simulink model "Trajectory_Tracking_Car_Backstepping_Algorithm"  (R2022b)
settings: Solver=FixedStepAuto  StartTime=0.0  StopTime=Tf  FixedStep=Ts  RelTol=1e-3
values from neighbouring files (symbols this model uses):
  alpha = 3    [Setup_Trajectory_FL_MPC.m]    (also in Setup_trajectory_Backstepping.m; Setup_trajectory_NL_MPC.m)
  alpha_c = 0.75    [Setup_trajectory_Backstepping.m]
  beta = 1.7    [Setup_Trajectory_FL_MPC.m]    (also in Setup_trajectory_Backstepping.m; Setup_trajectory_NL_MPC.m)
  d_x = 1    [Setup_trajectory_Backstepping.m]
  k3 = 1.65    [Setup_trajectory_Backstepping.m]
  l = 0.256    [Setup_Trajectory_FL_MPC.m]    (also in Setup_trajectory_Backstepping.m; Setup_trajectory_NL_MPC.m)
  N = 10    [Setup_Trajectory_FL_MPC.m]    (also in Setup_trajectory_Backstepping.m; Setup_trajectory_NL_MPC.m = 5)
  phi_max = 0.6    [Setup_trajectory_Backstepping.m]
  q0 = [x0;y0;theta0;phi0]    [Setup_Trajectory_FL_MPC.m]    (also in Setup_trajectory_Backstepping.m; Setup_trajectory_NL_MPC.m)
  sigma = 0.3    [Setup_trajectory_Backstepping.m]
  thetar = unwrap(atan2(ydr./v1r,xdr./v1r))    [Setup_Trajectory_FL_MPC.m]    (also in Setup_trajectory_Backstepping.m; Setup_trajectory_NL_MPC.m)
  Ts = 0.01    [Setup_Trajectory_FL_MPC.m]    (also in Setup_trajectory_Backstepping.m; Setup_trajectory_NL_MPC.m = 0.1)
  v1max = 2    [Setup_Trajectory_FL_MPC.m]    (also in Setup_trajectory_Backstepping.m; Setup_trajectory_NL_MPC.m)
libraries: simulink x3
settings Model: Creator=cricr  LastModifiedBy=user
settings SolverCC: AlgebraicLoopSolver=TrustRegion
settings DataIOCC: ReturnWorkspaceOutputs=off
settings DebuggingCC: UnconnectedInputMsg=warning  UnconnectedOutputMsg=warning  UnconnectedLineMsg=warning  SFMachineParentedDataDiag=warning  ArithmeticOperatorsInVariantConditions=warning
settings ModelReferenceCC: EnableRefExpFcnMdlSchedulingChecks=on
settings SFSimCC: SimUseLocalCustomCode=off  CustomCodeUndefinedFunction=UseInterfaceOnly
settings RTWCC: RTWUseLocalCustomCode=off

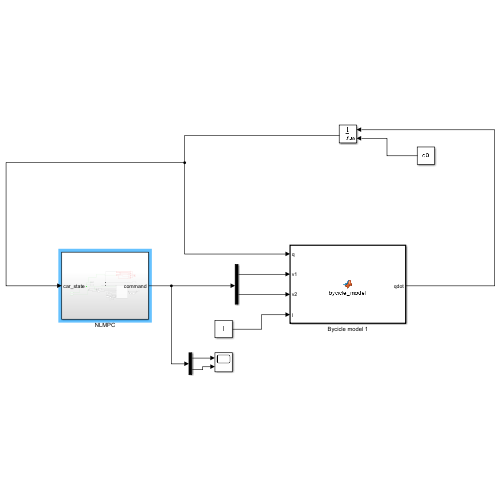
[thumbnail: Simulink's stored preview of the top-level diagram]
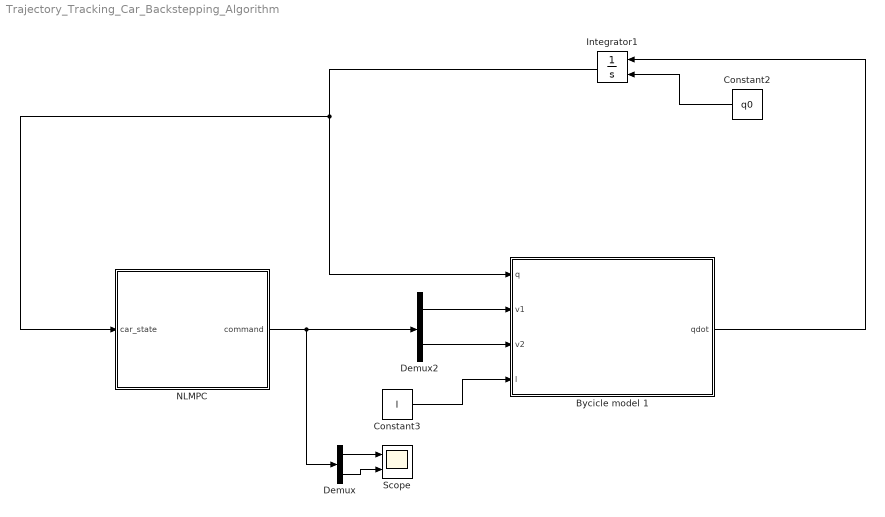
== system Trajectory_Tracking_Car_Backstepping_Algorithm ==
  Bycicle model 1 : MATLAB Function  TreatAsAtomicUnit=on
  Constant2 : Constant  Value=q0
  Constant3 : Constant  Value=l
  Demux : Demux  Outputs=2
  Demux2 : Demux  Outputs=2
  Integrator1 : Integrator  InitialConditionSource=external
  NLMPC : Subsystem
  Scope : Scope  NumInputPorts=2
  wires:
  Constant2/1 -> Integrator1/2
  Bycicle model 1/1(qdot) -> Integrator1/1
  Demux2/1 -> Bycicle model 1/2(v1)
  Demux2/2 -> Bycicle model 1/3(v2)
  Constant3/1 -> Bycicle model 1/4(l)
  Integrator1/1 -> NLMPC/1(car_state), Bycicle model 1/1(q)
  NLMPC/1(command) -> Demux/1, Demux2/1
  Demux/1 -> Scope/1
  Demux/2 -> Scope/2

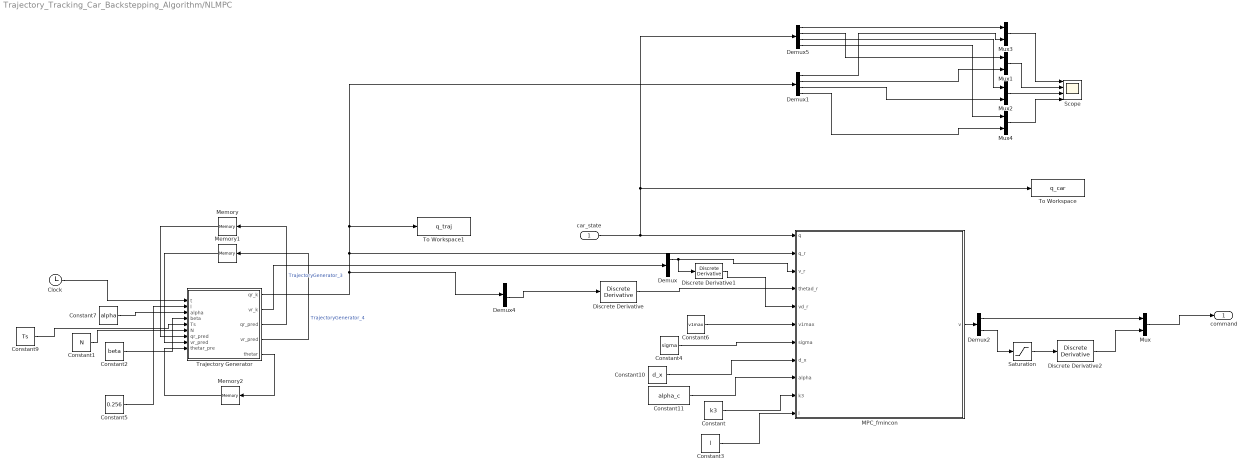
== system Trajectory_Tracking_Car_Backstepping_Algorithm/NLMPC ==
  car_state : Inport
  Clock : Clock
  Constant : Constant  Value=k3
  Constant1 : Constant  Value=N
  Constant10 : Constant  Value=d_x
  Constant11 : Constant  Value=alpha_c
  Constant2 : Constant  Value=beta
  Constant3 : Constant  Value=l
  Constant4 : Constant  Value=sigma
  Constant5 : Constant  Value=0.256
  Constant6 : Constant  Value=v1max
  Constant7 : Constant  Value=alpha
  Constant9 : Constant  Value=Ts
  Demux : Demux  Outputs=2
  Demux1 : Demux
  Demux2 : Demux  Outputs=2
  Demux4 : Demux
  Demux5 : Demux
  Discrete Derivative : simulink/Discrete/Discrete Derivative  gainval=1.0  ICPrevScaledInput=0.0  OutMin=[]  OutMax=[]  OutDataType=fixdt(1, 16)  OutScaling=2^-10  DoSatur=off
  Discrete Derivative1 : simulink/Discrete/Discrete Derivative  gainval=1.0  ICPrevScaledInput=0.0  OutMin=[]  OutMax=[]  OutDataType=fixdt(1, 16)  OutScaling=2^-10  DoSatur=off
  Discrete Derivative2 : simulink/Discrete/Discrete Derivative  gainval=1.0  ICPrevScaledInput=0.0  OutMin=[]  OutMax=[]  OutDataType=fixdt(1, 16)  OutScaling=2^-10  DoSatur=off
  MPC_fmincon : MATLAB Function  TreatAsAtomicUnit=on
  Memory : Memory  InitialCondition=zeros(4,N)
  Memory1 : Memory  InitialCondition=zeros(2,N)
  Memory2 : Memory  InitialCondition=thetar(1)
  Mux{,1..4} (5 alike) : Mux  Inputs=2
  Saturation : Saturate  UpperLimit=phi_max  LowerLimit=-phi_max  LinearizeAsGain=off
  Scope : Scope  NumInputPorts=4
  To Workspace : ToWorkspace  VariableName=q_car  SaveFormat=Timeseries  SampleTime=-1
  To Workspace1 : ToWorkspace  VariableName=q_traj  SaveFormat=Timeseries  SampleTime=-1
      settings: Save2DSignal=2-D array (concatenate along first dimension)
  Trajectory Generator : MATLAB Function  TreatAsAtomicUnit=on
  command : Outport
  wires:
  Demux5/2 -> Mux1/1
  Demux5/4 -> Mux4/1
  Mux2/1 -> Scope/3
  Mux3/1 -> Scope/1
  Constant10/1 -> MPC_fmincon/8(d_x)
  Demux1/3 -> Mux2/2
  Mux1/1 -> Scope/2
  Demux1/4 -> Mux4/2
  Mux4/1 -> Scope/4
  Demux5/1 -> Mux3/1
  car_state/1 -> MPC_fmincon/1(q), Demux5/1, To Workspace/1
  Demux1/1 -> Mux3/2
  Demux1/2 -> Mux1/2
  Demux5/3 -> Mux2/1
  Constant4/1 -> MPC_fmincon/7(sigma)
  Constant6/1 -> MPC_fmincon/6(v1max)
  Mux/1 -> command/1
  MPC_fmincon/1(v) -> Demux2/1
  Demux2/2 -> Saturation/1
  Saturation/1 -> Discrete Derivative2/1
  Discrete Derivative2/1 -> Mux/2
  Demux2/1 -> Mux/1
  Constant3/1 -> MPC_fmincon/11(l)
  Constant11/1 -> MPC_fmincon/9(alpha)
  Constant/1 -> MPC_fmincon/10(k3)
  Demux/1 -> Discrete Derivative1/1, MPC_fmincon/3(v_r)
  Demux4/3 -> Discrete Derivative/1
  Discrete Derivative/1 -> MPC_fmincon/4(thetad_r)
  Discrete Derivative1/1 -> MPC_fmincon/5(vd_r)
  Constant7/1 -> Trajectory Generator/3(alpha)
  Constant9/1 -> Trajectory Generator/5(Ts)
  Constant5/1 -> Trajectory Generator/2(l)
  Memory1/1 -> Trajectory Generator/8("vr_pred ")
  Trajectory Generator/3(qr_pred) -> Memory/1  "TrajectoryGenerator_3"
  Clock/1 -> Trajectory Generator/1(t)
  Constant1/1 -> Trajectory Generator/6(N)
  Trajectory Generator/5(thetar) -> Memory2/1
  Trajectory Generator/4(vr_pred) -> Memory1/1  "TrajectoryGenerator_4"
  Constant2/1 -> Trajectory Generator/4(beta)
  Memory/1 -> Trajectory Generator/7("qr_pred ")
  Memory2/1 -> Trajectory Generator/9(thetar_pre)
  Trajectory Generator/2(vr_k) -> Demux/1
  Trajectory Generator/1(qr_k) -> MPC_fmincon/2(q_r), Demux1/1, To Workspace1/1, Demux4/1

== matlab function Trajectory_Tracking_Car_Backstepping_Algorithm/NLMPC/MPC_fmincon ==
  data: q input; v output; q_r input; v_r input; thetad_r input; vd_r input; v1max input; sigma input; d_x input; alpha input; k3 input; l input
function v = Zhang_tracking_controller(q,q_r,v_r,thetad_r,vd_r,v1max,sigma,d_x,alpha,k3,l)



if v_r==0
    v_r=0.0001;
end

x=q(1); y=q(2); theta=q(3); 
x_r=q_r(1); y_r=q_r(2); theta_r=q_r(3); 


q_e=[cos(theta) sin(theta) 0 ;
    -sin(theta) cos(theta) 0;
    0 0 1]*[x_r-x; y_r-y; theta_r-theta];


x_e=q_e(1); y_e=q_e(2); theta_e=q_e(3); 



Delta=v1max-v_r*tanh(v_r/sigma);


if abs(x_e)<=d_x
    k1=-Delta/(2*d_x^3)*abs(x_e)^2+3*Delta/(2*d_x);
else
    k1=Delta/abs(x_e);
end


u1=v_r*cos(theta_e)+k1*x_e;



k2=alpha*v_r;

y_e_tilde=y_e+k2/v_r*sin(theta_e);

u2_star=(k3*y_e_tilde+2*v_r*sin(theta_e)+k2/v_r*cos(theta_e)*thetad_r-k2/v_r^2*sin(theta_r)*vd_r)/(x_e+k2/v_r*cos(theta_e));

u2=atan(l/u1*u2_star);


v=[u1;u2];

end

== matlab function Trajectory_Tracking_Car_Backstepping_Algorithm/NLMPC/Trajectory Generator ==
  data: t input; qr_k output; vr_k output; l input; alpha input; beta input; Ts input; qr_pred output size=[4 N]; vr_pred output size=[2 N]; N input; qr_pred input; vr_pred input; thetar_pre input; thetar output
function [qr_k,vr_k,qr_pred, vr_pred,thetar] = Trajectory(t,l,alpha,beta,Ts,N,qr_pred,vr_pred,thetar_pre)




xr=alpha*sin(t/beta);
yr=alpha*sin(t/(2*beta));

xdr=alpha*cos(t/beta)*(1/(beta));
ydr=alpha*cos(t/(2*beta))*(1/(2*beta));


xddr=-alpha*sin(t/beta)*(1/(beta))^2;
yddr=-alpha*sin(t/(2*beta))*(1/(2*beta))^2;

xdddr=-alpha*cos(t/beta)*(1/(beta))^3;
ydddr=-alpha*cos(t/(2*beta))*(1/(2*beta))^3;

%Driving velocity reference
v1r=sqrt(xdr^2+ydr^2); %Linear velocity of the trajectory


thetar=atan2(ydr/v1r,xdr/v1r);

theta=[thetar_pre thetar];

theta=unwrap(theta);
thetar=theta(2);


%Steering angle reference
phir=atan(l*(yddr*xdr-xddr*ydr)/v1r^3);

%Steering velocity reference
v2r=l*v1r*((ydddr*xdr-xdddr*ydr)*v1r^2-3*(yddr*xdr-xddr*ydr)*(xdr*xddr+ydr*yddr))/(v1r^6+l^2*(yddr*xdr-xddr*ydr)^2);


qr_k=[xr;yr;thetar;phir];
vr_k=[v1r;v2r];


for i=1:N
    t=t+(i-1)*Ts;
    xr=alpha*sin(t/beta);
    yr=alpha*sin(t/(2*beta));

    xdr=alpha*cos(t/beta)*(1/(beta));
    ydr=alpha*cos(t/(2*beta))*(1/(2*beta));


    xddr=-alpha*sin(t/beta)*(1/(beta))^2;
    yddr=-alpha*sin(t/(2*beta))*(1/(2*beta))^2;

    xdddr=-alpha*cos(t/beta)*(1/(beta))^3;
    ydddr=-alpha*cos(t/(2*beta))*(1/(2*beta))^3;



    %Driving velocity reference
    v1r=sqrt(xdr^2+ydr^2); %Linear velocity of the trajectory

    

    thetar=atan2(ydr/v1r,xdr/v1r);

    if i==1
        theta=[thetar_pre thetar];
        theta=unwrap(theta);
        thetar=theta(2);
        thetar_pre=thetar;

    else
       
        theta=[thetar_pre thetar];
        theta=unwrap(theta);
        thetar=theta(2);


    end


    %Steering angle reference
    phir=atan(l*(yddr*xdr-xddr*ydr)/v1r^3);

    %Steering velocity reference
    v2r=l*v1r*((ydddr*xdr-xdddr*ydr)*v1r^2-3*(yddr*xdr-xddr*ydr)*(xdr*xddr+ydr*yddr))/(v1r^6+l^2*(yddr*xdr-xddr*ydr)^2);



    %Nonlinear model reference state
    qr_pred(:,i)=[xr;yr;thetar;phir];
    vr_pred(:,i)=[v1r;v2r];

end

 qr_pred(3,:)= unwrap(qr_pred(3,:));

== matlab function Trajectory_Tracking_Car_Backstepping_Algorithm/Bycicle model 1 ==
  data: q input; qdot output; v1 input; v2 input; l input
function qdot  = bycicle_model(q,v1,v2,l)

%This function implements the car kinematic model
x=q(1);
y=q(2);
theta=q(3);
phi=q(4);

q1dot=v1*cos(theta);
q2dot=v1*sin(theta);
q3dot = v1*tan(phi)/l;
q4dot = v2;


qdot= [q1dot;q2dot;q3dot;q4dot];
end
